simulink model "LDPC_sim"  (R2024a)
settings: Solver=VariableStepDiscrete  StartTime=0.0  StopTime=inf  RelTol=1e-3  EnableMultiTasking=on
PreLoadFcn:
  | N = 7;    % Codeword length
  | EbNo = 8; % Default EbNo
  | K = 4;    % Message length
libraries: commdigbbndpm3 x2, commblkcod2 x2, commrandsrc3 x1, commchan3 x1, commsink2 x1
(part 20 of 20)

== system LDPC_sim/Subsystem ==
